simulink model "test_num"  (Simulink 8.7)
settings: Solver=ode3  StartTime=0.0  StopTime=2  FixedStep=Step_Time  MaxStep=Step_Time  RelTol=1e-3
values from neighbouring files (symbols this model uses):
  q0 = homeConfiguration(robot)    [inv_example.m]
settings Model: Creator=saeed  LastModifiedBy=S.Mansouri
settings DataIOCC: SignalLoggingSaveFormat=ModelDataLogs
settings OptimizationCC: ExpressionDepthLimit=2147483647
settings DebuggingCC: SolverPrmCheckMsg=warning  FcnCallInpInsideContextMsg=UseLocalSettings  StateNameClashWarn=warning
settings GRTTargetCC: CombineOutputUpdateFcns=off  GRTInterface=on

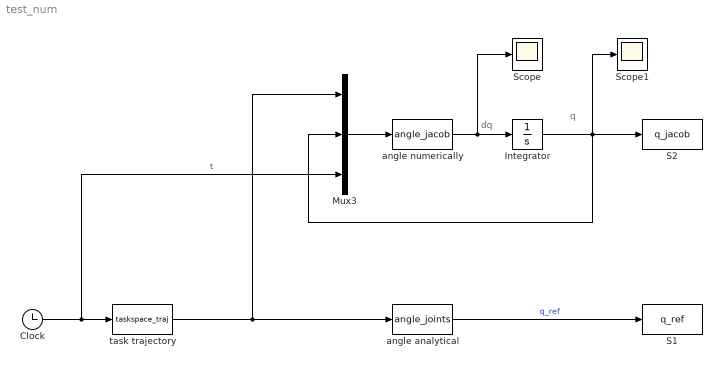
== system test_num ==
  note: dq
  note: q
  Clock : Clock
  Integrator : Integrator  InitialCondition=q0
  Mux3 : Mux  Inputs=3
  S1 : ToWorkspace  VariableName=q_ref  SaveFormat=Structure With Time  SampleTime=-1
  S2 : ToWorkspace  VariableName=q_jacob  SaveFormat=Structure With Time  SampleTime=-1
  Scope : Scope
  Scope1 : Scope
  angle analytical : MATLABFcn  MATLABFcn=angle_joints
  angle numerically : MATLABFcn  MATLABFcn=angle_jacob
  task trajectory : MATLABFcn  MATLABFcn=taskspace_traj
  wires:
  Clock/1 -> Mux3/3, task trajectory/1  "t"
  angle analytical/1 -> S1/1  "q_ref"
  task trajectory/1 -> angle analytical/1, Mux3/1
  Mux3/1 -> angle numerically/1
  angle numerically/1 -> Integrator/1, Scope/1
  Integrator/1 -> Mux3/2, S2/1, Scope1/1
